simulink model "AircraftSimulation_RealTime1a"  (R2017a)
settings: Solver=ode45  StartTime=0.0  StopTime=inf  RelTol=1e-3  EnableMultiTasking=on
model workspace (MAT data in the model file):
  MCOS : class17 (value not decoded)
values from neighbouring files (symbols this model uses):
  AR = 9.8    [ControlTuning.m]
  b = 12.8016    [ControlTuning.m]
  c = 1.3533    [ControlTuning.m]
  D = d    [rscale.m]
  m = 2521    [ControlTuning.m]
  N = inv([A,B;C,D])*Z'    [rscale.m]
  rho = 0.66    [ControlTuning.m]
  S = 16.72254    [ControlTuning.m]
  s = tf('s')    [ControlTuning.m]    (also in rscale.m = size(A,1))
  W = m*g    (= 24731.01)    [ControlTuning.m]
  Z = [zeros([1,s]) 1]    [rscale.m]
  zeta = Ix*Iz - Ixz^2    (= 5250689.81)    [ControlTuning.m]
undefined symbols (not defined in the file or in its folder): cdo, CLa, ClB, Clda, CLde, Cldr, CLmax, CLo, Clp, CLq, Clr, Cma, Cmde, Cmo, Cmq, CnB, Cnda, Cndr, Cnp, Cnr, CYB, CYda, CYdr, CYp, CYr, da, de, dr, dT, dV_x, dV_y, dV_z, elevation, h, I, Isp, L, mo, mu_e, springK, StallAngle, T, tblackstrip, tControl, tWind, X, xground, xland, Y, yground, yland, ZeroTolerance
libraries: sm_lib x51, nesl_utility x18, simulink x10, realtime_pacer_lib x1
(part 2 of 2)

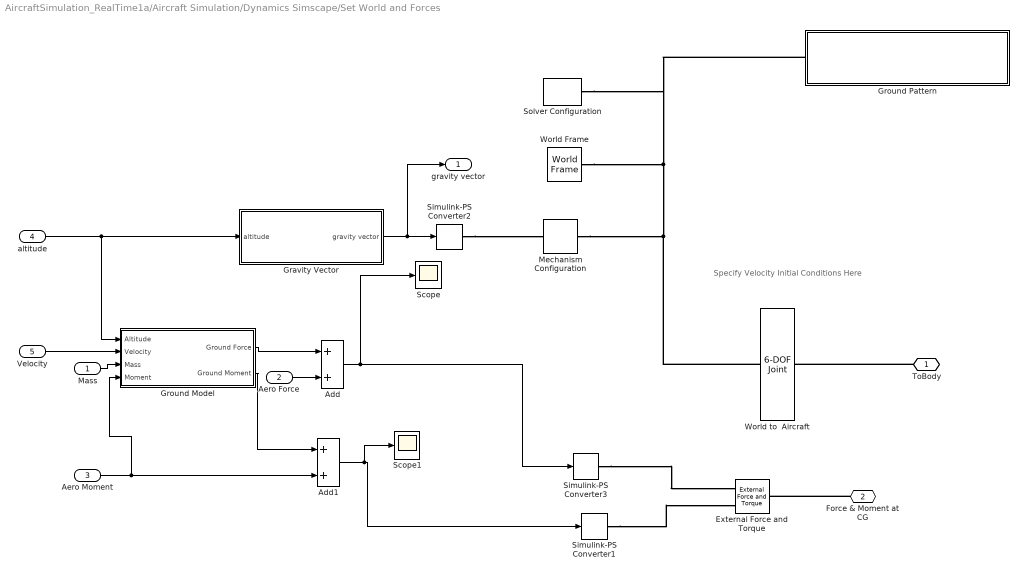
== system AircraftSimulation_RealTime1a/Aircraft Simulation/Dynamics Simscape/Set World and Forces ==
  note: Specify Velocity Initial Conditions Here
  Mass : Inport
  Aero Force : Inport  Port=2
  Aero Moment : Inport  Port=3
  altitude : Inport  Port=4
  Velocity : Inport  Port=5
  Add : Sum
  Add1 : Sum
  External Force and Torque : sm_lib/Forces and Torques/External Force and Torque  ForceResolutionFrame=AttachedFrame  EnableForceX=off  EnableForceY=off  EnableForceZ=off  EnableForce=on  TorqueResolutionFrame=AttachedFrame  EnableTorqueX=off  EnableTorqueY=off  EnableTorqueZ=off  EnableTorque=on
  Gravity Vector : Subsystem
  Ground Model : Subsystem
  Ground Pattern : Subsystem
  Mechanism Configuration : sm_lib/Utilities/Mechanism Configuration  UniformGravity=TimeVarying  GravityVector=[0 0 -9.80665]  GravityUnits=m/s^2  LinearizationDelta=0.001
  Scope : Scope
  Scope1 : Scope
  Simulink-PS Converter1 : nesl_utility/Simulink-PS Converter  PhysicalDomain=network_engine_domain  SubClassName=ps_input  LeftPortType=input  RightPortType=output  PseudoPeriodic=off  Frequencies=[]  NoiseDistribution=none  NoiseParameters=[]  Unit=1  AffineConversion=off  FilteringAndDerivatives=provide  SimscapeFilterOrder=1  InputFilterTimeConstant=0.001  UdotUserProvided=0
  Simulink-PS Converter2 : nesl_utility/Simulink-PS Converter  PhysicalDomain=network_engine_domain  SubClassName=ps_input  LeftPortType=input  RightPortType=output  PseudoPeriodic=off  Frequencies=[]  NoiseDistribution=none  NoiseParameters=[]  Unit=1  AffineConversion=off  FilteringAndDerivatives=provide  SimscapeFilterOrder=1  InputFilterTimeConstant=0.001  UdotUserProvided=0
  Simulink-PS Converter3 : nesl_utility/Simulink-PS Converter  PhysicalDomain=network_engine_domain  SubClassName=ps_input  LeftPortType=input  RightPortType=output  PseudoPeriodic=off  Frequencies=[]  NoiseDistribution=none  NoiseParameters=[]  Unit=1  AffineConversion=off  FilteringAndDerivatives=provide  SimscapeFilterOrder=1  InputFilterTimeConstant=0.001  UdotUserProvided=0
  Solver Configuration : nesl_utility/Solver Configuration  PhysicalDomain=network_engine_domain  SubClassName=solver  LeftPortType=input  RightPortType=generic  Accelerate=off  Tones=[]  Harmonics=[]  SimulateNoise=off  Profile=off  UseLocalSampling=off  EnableSwitchedLinearOptims=on  FrequencyDomain=off  UseCCode=off  RelTol=0.001  AbsTol=1e-06  MinStep=1e-09  ToWorkspace=off  RevertToSquareIcSolve=off  NumHomotopyIterations=100  PhasorMode=off  PhasorModeNumHarmonics=1  OverrideAbsTol=off  DoDC=off  ResidualTolerance=1e-09  UseLocalSolver=off  LocalSolverChoice=NE_BACKWARD_EULER_ADVANCER  LocalSolverSampleTime=0.001  DoFixedCost=off  MaxNonlinIter=3  MaxModeIter=2  LinearAlgebra=Sparse  DelaysMemoryBudget=1024  AutomaticFiltering=on  FilteringTimeConstant=0.001
  World Frame : sm_lib/Frames and Transforms/World Frame
  World to  Aircraft : sm_lib/Joints/6-DOF Joint  SenseConstraintForce=off  SenseConstraintForceX=off  SenseConstraintForceY=off  SenseConstraintForceZ=off  SenseConstraintTorque=off  SenseConstraintTorqueX=off  SenseConstraintTorqueY=off  SenseConstraintTorqueZ=off  SenseTotalForce=off  SenseTotalForceX=off  SenseTotalForceY=off  SenseTotalForceZ=off  SenseTotalTorque=off  SenseTotalTorqueX=off  SenseTotalTorqueY=off  SenseTotalTorqueZ=off  CompositeWrenchDir=BaseOnFollower  CompositeWrenchFrame=BaseFrame  PxEquilibriumPosition=0  PxEquilibriumPositionUnits=m  PxSpringStiffness=0  PxSpringStiffnessUnits=N/m  PxDampingCoefficient=0  PxDampingCoefficientUnits=N/(m/s)  PxTorqueActuationMode=NoTorque  PxMotionActuationMode=ComputedMotion  PxSensePosition=off  PxSenseVelocity=off  PxSenseAcceleration=off  PxSenseTorqueForce=off  PxPositionTargetSpecify=on  PxPositionTargetPriority=High  PxPositionTargetValue=x_initial  PxPositionTargetValueUnits=m  PxVelocityTargetSpecify=on  PxVelocityTargetPriority=High  PxVelocityTargetValue=u_inertial  PxVelocityTargetValueUnits=m/s  PyEquilibriumPosition=0  PyEquilibriumPositionUnits=m  PySpringStiffness=0  PySpringStiffnessUnits=N/m  PyDampingCoefficient=0  PyDampingCoefficientUnits=N/(m/s)  PyTorqueActuationMode=NoTorque  PyMotionActuationMode=ComputedMotion  PySensePosition=off  PySenseVelocity=off  PySenseAcceleration=off  PySenseTorqueForce=off  PyPositionTargetSpecify=on  PyPositionTargetPriority=High  PyPositionTargetValue=y_initial  PyPositionTargetValueUnits=m  PyVelocityTargetSpecify=on  PyVelocityTargetPriority=High  PyVelocityTargetValue=v_inertial  PyVelocityTargetValueUnits=m/s  PzEquilibriumPosition=0  PzEquilibriumPositionUnits=m  PzSpringStiffness=0  PzSpringStiffnessUnits=N/m  PzDampingCoefficient=0  PzDampingCoefficientUnits=N/(m/s)  PzTorqueActuationMode=NoTorque  PzMotionActuationMode=ComputedMotion  PzSensePosition=off  PzSenseVelocity=off  PzSenseAcceleration=off  PzSenseTorqueForce=off  PzPositionTargetSpecify=on  PzPositionTargetPriority=High  PzPositionTargetValue=alt  PzPositionTargetValueUnits=m  PzVelocityTargetSpecify=on  PzVelocityTargetPriority=High  PzVelocityTargetValue=w_inertial  PzVelocityTargetValueUnits=m/s  SphDefPosRotationMethod=None  SphDefPosRotationAngleUnits=deg  SphDefPosRotationStandardAxis=+Z  SphDefPosRotationAngle=0.0  SphDefPosRotationArbitraryAxis=[0 0 1]  SphDefPosFollAlignAxisA=+X  SphDefPosBaseAlignAxisA=+Y  SphDefPosFollAlignAxisB=+Y  SphDefPosBaseAlignAxisB=+Z  SphDefPosRotationSequenceAxes=FollowerAxes  SphDefPosRotationSequence=XYX  SphDefPosRotationSequenceAngles=[0 0 0]  SphDefPosRotationSequenceAnglesUnits=deg  SphDefPosRotationMatrix=[1 0 0; 0 1 0; 0 0 1]  SphEqPosRotationMethod=None  SphEqPosRotationAngleUnits=deg  SphEqPosRotationStandardAxis=+Z  SphEqPosRotationAngle=0.0  SphEqPosRotationArbitraryAxis=[0 0 1]  SphEqPosFollAlignAxisA=+X  SphEqPosBaseAlignAxisA=+Y  SphEqPosFollAlignAxisB=+Y  SphEqPosBaseAlignAxisB=+Z  SphEqPosRotationSequenceAxes=FollowerAxes  SphEqPosRotationSequence=XYX  SphEqPosRotationSequenceAngles=[0 0 0]  SphEqPosRotationSequenceAnglesUnits=deg  SphEqPosRotationMatrix=[1 0 0; 0 1 0; 0 0 1]  SphSpringStiffness=0  SphSpringStiffnessUnits=N*m/deg  SphDampingCoefficient=0  SphDampingCoefficientUnits=N*m/(deg/s)  SphActuateTorqueX=off  SphActuateTorqueY=off  SphActuateTorqueZ=off  SphActuateTorque=on  SphTorqueActuationMode=NoTorque  SphMotionActuationMode=ComputedMotion  SphActuationFrame=BaseFrame  SphSensePosition=off  SphSenseVelocityX=off  SphSenseVelocityY=off  SphSenseVelocityZ=off  SphSenseVelocity=off  SphSenseAccelerationX=off  SphSenseAccelerationY=off  SphSenseAccelerationZ=off  SphSenseAcceleration=off  SphSenseTorqueX=off  SphSenseTorqueY=off  SphSenseTorqueZ=off  SphSenseTorqueForce=off  SphSensingFrame=BaseFrame  SphPositionTargetRotationMethod=StandardAxis  SphPositionTargetRotationAngleUnits=deg  SphPositionTargetRotationStandardAxis=+Y  SphPositionTargetRotationAngle=pitch_initial  SphPositionTargetRotationArbitraryAxis=[0 0 1]  SphPositionTargetFollAlignAxisA=+X  SphPositionTargetBaseAlignAxisA=+Y  SphPositionTargetFollAlignAxisB=+Y  SphPositionTargetBaseAlignAxisB=+Z  SphPositionTargetRotationSequenceAxes=FollowerAxes  SphPositionTargetRotationSequence=XYX  SphPositionTargetRotationSequenceAngles=[0 0 0]  SphPositionTargetRotationSequenceAnglesUnits=deg  SphPositionTargetRotationMatrix=[1 0 0; 0 1 0; 0 0 1]  SphPositionTargetSpecify=on  SphPositionTargetPriority=High  SphVelocityTargetValue=[0 0 0]  SphVelocityTargetValueUnits=deg/s  SphVelocityTargetSpecify=off  SphVelocityTargetPriority=High  SphVelocityTargetInFollowerFrame=on
  ToBody : PMIOPort  Port=1  Side=Right
  Force & Moment at CG : PMIOPort  Port=2  Side=Right
  gravity vector : Outport
  wires:
  Gravity Vector/1(gravity vector) -> gravity vector/1, Simulink-PS Converter2/1
  altitude/1 -> Ground Model/1(Altitude), Gravity Vector/1(altitude)
  Velocity/1 -> Ground Model/2(Velocity)
  Mass/1 -> Ground Model/3(Mass)
  Ground Model/1(Ground Force) -> Add/1
  Aero Force/1 -> Add/2
  Add/1 -> Scope/1, Simulink-PS Converter3/1
  Aero Moment/1 -> Ground Model/4(Moment), Add1/2
  Add1/1 -> Scope1/1, Simulink-PS Converter1/1
  Ground Model/2(Ground Moment) -> Add1/1
  connections:
  Simulink-PS Converter2/RConn1 -- Mechanism Configuration/LConn1
  Ground Pattern/LConn1 -- Solver Configuration/RConn1 -- World to  Aircraft/LConn1 -- Mechanism Configuration/RConn1 -- World Frame/RConn1
  ToBody/RConn1 -- World to  Aircraft/RConn1
  Simulink-PS Converter3/RConn1 -- External Force and Torque/LConn1
  Simulink-PS Converter1/RConn1 -- External Force and Torque/LConn2
  Force & Moment at CG/RConn1 -- External Force and Torque/RConn1

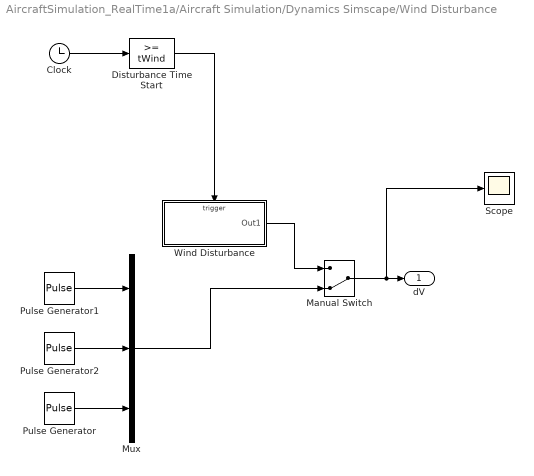
== system AircraftSimulation_RealTime1a/Aircraft Simulation/Dynamics Simscape/Wind Disturbance ==
  Clock : Clock
  Disturbance Time Start : simulink/Logic and Bit Operations/Compare To Constant  relop=>=  const=tWind  OutDataTypeStr=boolean
  Manual Switch : ManualSwitch  CurrentSetting=0
  Mux : Mux  Inputs=3
  Pulse Generator : DiscretePulseGenerator  PulseType=Time based  Amplitude=dV_z  Period=250  PulseWidth=.5  PhaseDelay=5
  Pulse Generator1 : DiscretePulseGenerator  PulseType=Time based  Amplitude=dV_x  Period=250  PulseWidth=.5  PhaseDelay=5
  Pulse Generator2 : DiscretePulseGenerator  PulseType=Time based  Amplitude=dV_y  Period=250  PulseWidth=.5  PhaseDelay=5
  Scope : Scope
  "Wind Disturbance " : Subsystem  TreatAsAtomicUnit=on
  dV : Outport
  wires:
  Clock/1 -> Disturbance Time Start/1
  Disturbance Time Start/1 -> "Wind Disturbance "/Trigger
  Manual Switch/1 -> Scope/1, dV/1
  "Wind Disturbance "/1(Out1) -> Manual Switch/1
  Pulse Generator/1 -> Mux/3
  Mux/1 -> Manual Switch/2
  Pulse Generator2/1 -> Mux/2
  Pulse Generator1/1 -> Mux/1

== system AircraftSimulation_RealTime1a/Aircraft Simulation/Flight Command/Command disturbance ==
  Clock : Clock
  "Cmd Disturbance " : Subsystem  TreatAsAtomicUnit=on
  Disturbance Time Start : simulink/Logic and Bit Operations/Compare To Constant  relop=>=  const=tControl  OutDataTypeStr=boolean
  dCmd : Outport
  wires:
  Clock/1 -> Disturbance Time Start/1
  Disturbance Time Start/1 -> "Cmd Disturbance "/Trigger
  "Cmd Disturbance "/1(Out1) -> dCmd/1

== system AircraftSimulation_RealTime1a/Aircraft Simulation/Aerodynamics Simscape/Forces and Moments/Small Number = Zero6 ==
  In1 : Inport
  Abs : Abs
  Compare To Constant : simulink/Logic and Bit Operations/Compare To Constant  relop=>=  const=ZeroTolerance  OutDataTypeStr=boolean
  Product1 : Product  Inputs=3
  Sign : Signum
  Out1 : Outport
  wires:
  Sign/1 -> Product1/3
  Abs/1 -> Compare To Constant/1, Product1/1
  Product1/1 -> Out1/1
  Compare To Constant/1 -> Product1/2
  In1/1 -> Abs/1, Sign/1

== system AircraftSimulation_RealTime1a/Aircraft Simulation/Aerodynamics Simscape/Forces and Moments/Stall ==
  In1 : Inport
  Abs : Abs
  Compare To Constant : simulink/Logic and Bit Operations/Compare To Constant  relop=>  const=StallAngle  OutDataTypeStr=boolean
  Demux : Demux
  Terminator : Terminator
  Terminator1 : Terminator
  Terminator2 : Terminator
  Stall : Outport
  wires:
  Demux/3 -> Terminator1/1
  Demux/4 -> Terminator2/1
  Demux/2 -> Abs/1
  Demux/1 -> Terminator/1
  Compare To Constant/1 -> Stall/1
  In1/1 -> Demux/1
  Abs/1 -> Compare To Constant/1

== system AircraftSimulation_RealTime1a/Aircraft Simulation/Aerodynamics Simscape/Forces and Moments/stall effect ==
  lift : Inport
  stall : Inport  Port=2
  Compare To Constant : simulink/Logic and Bit Operations/Compare To Constant  relop=<=  const=1  OutDataTypeStr=boolean
  Product1 : Product
  Lift : Outport
  wires:
  lift/1 -> Product1/1
  Compare To Constant/1 -> Product1/2
  stall/1 -> Compare To Constant/1
  Product1/1 -> Lift/1

== system AircraftSimulation_RealTime1a/Aircraft Simulation/Aerodynamics Simscape/Forces and Moments/stall effect1 ==
  moment : Inport
  stall : Inport  Port=2
  Compare To Constant : simulink/Logic and Bit Operations/Compare To Constant  relop=<=  const=1  OutDataTypeStr=boolean
  Product1 : Product
  Moment : Outport
  wires:
  Product1/1 -> Moment/1
  stall/1 -> Compare To Constant/1
  Compare To Constant/1 -> Product1/2
  moment/1 -> Product1/1

== system AircraftSimulation_RealTime1a/Aircraft Simulation/Dynamics Simscape/Derived States/Cannot Divide By Zero ==
  Denominator In : Inport
  Else Action Subsystem : Subsystem  TreatAsAtomicUnit=on
  If : If  IfExpression=u1 == 0
  "If Action Subsystem " : Subsystem  TreatAsAtomicUnit=on
  Merge : Merge
  Denominator Out : Outport
  wires:
  Denominator In/1 -> Else Action Subsystem/1(In1), If/1
  "If Action Subsystem "/1(Out1) -> Merge/1
  If/1 -> "If Action Subsystem "/Action
  If/2 -> Else Action Subsystem/Action
  Else Action Subsystem/1(Out1) -> Merge/2
  Merge/1 -> Denominator Out/1

== system AircraftSimulation_RealTime1a/Aircraft Simulation/Dynamics Simscape/Derived States/Cannot Divide By Zero1 ==
  Denominator In : Inport
  Else Action Subsystem : Subsystem  TreatAsAtomicUnit=on
  If : If  IfExpression=u1 == 0
  "If Action Subsystem " : Subsystem  TreatAsAtomicUnit=on
  Merge : Merge
  Denominator Out : Outport
  wires:
  Merge/1 -> Denominator Out/1
  Else Action Subsystem/1(Out1) -> Merge/2
  If/2 -> Else Action Subsystem/Action
  If/1 -> "If Action Subsystem "/Action
  "If Action Subsystem "/1(Out1) -> Merge/1
  Denominator In/1 -> If/1, Else Action Subsystem/1(In1)

== system AircraftSimulation_RealTime1a/Aircraft Simulation/Dynamics Simscape/Derived States/Magnitude ==
  Vector : Inport
  Demux : Demux  Outputs=3
  Product1 : Product
  Product2 : Product
  Product3 : Product
  Sqrt : Sqrt  SaturateOnIntegerOverflow=on
  Sum : Sum  Inputs=+++
  Magnitude : Outport
  wires:
  Demux/1 -> Product1/1, Product1/2
  Demux/3 -> Product3/1, Product3/2
  Product2/1 -> Sum/2
  Product1/1 -> Sum/1
  Sum/1 -> Sqrt/1
  Demux/2 -> Product2/1, Product2/2
  Product3/1 -> Sum/3
  Vector/1 -> Demux/1
  Sqrt/1 -> Magnitude/1

== system AircraftSimulation_RealTime1a/Aircraft Simulation/Dynamics Simscape/Derived States/Small Number = Zero1 ==
  In1 : Inport
  Abs : Abs
  Compare To Constant : simulink/Logic and Bit Operations/Compare To Constant  relop=>=  const=ZeroTolerance  OutDataTypeStr=boolean
  Product1 : Product  Inputs=3
  Sign : Signum
  Out1 : Outport
  wires:
  In1/1 -> Sign/1, Abs/1
  Compare To Constant/1 -> Product1/2
  Product1/1 -> Out1/1
  Abs/1 -> Product1/1, Compare To Constant/1
  Sign/1 -> Product1/3

== system AircraftSimulation_RealTime1a/Aircraft Simulation/Dynamics Simscape/Derived States/Small Number = Zero2 ==
  In1 : Inport
  Abs : Abs
  Compare To Constant : simulink/Logic and Bit Operations/Compare To Constant  relop=>=  const=ZeroTolerance  OutDataTypeStr=boolean
  Product1 : Product  Inputs=3
  Sign : Signum
  Out1 : Outport
  wires:
  In1/1 -> Sign/1, Abs/1
  Compare To Constant/1 -> Product1/2
  Product1/1 -> Out1/1
  Abs/1 -> Product1/1, Compare To Constant/1
  Sign/1 -> Product1/3

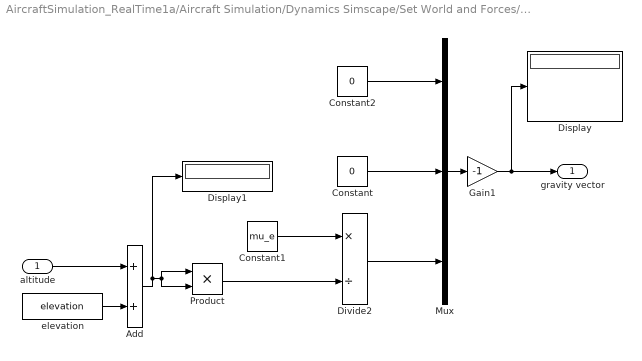
== system AircraftSimulation_RealTime1a/Aircraft Simulation/Dynamics Simscape/Set World and Forces/Gravity Vector ==
  altitude : Inport
  Add : Sum
  Constant : Constant  Value=0
  Constant1 : Constant  Value=mu_e
  Constant2 : Constant  Value=0
  Display : Display
  Display1 : Display
  Divide2 : Product  Inputs=*/
  Gain1 : Gain  Gain=-1
  Mux : Mux  Inputs=3
  Product : Product
  elevation : Constant  Value=elevation
  gravity vector : Outport
  wires:
  Constant1/1 -> Divide2/1
  Constant/1 -> Mux/2
  Product/1 -> Divide2/2
  Add/1 -> Display1/1, Product/1, Product/2
  elevation/1 -> Add/2
  Constant2/1 -> Mux/1
  Mux/1 -> Gain1/1
  Divide2/1 -> Mux/3
  altitude/1 -> Add/1
  Gain1/1 -> Display/1, gravity vector/1

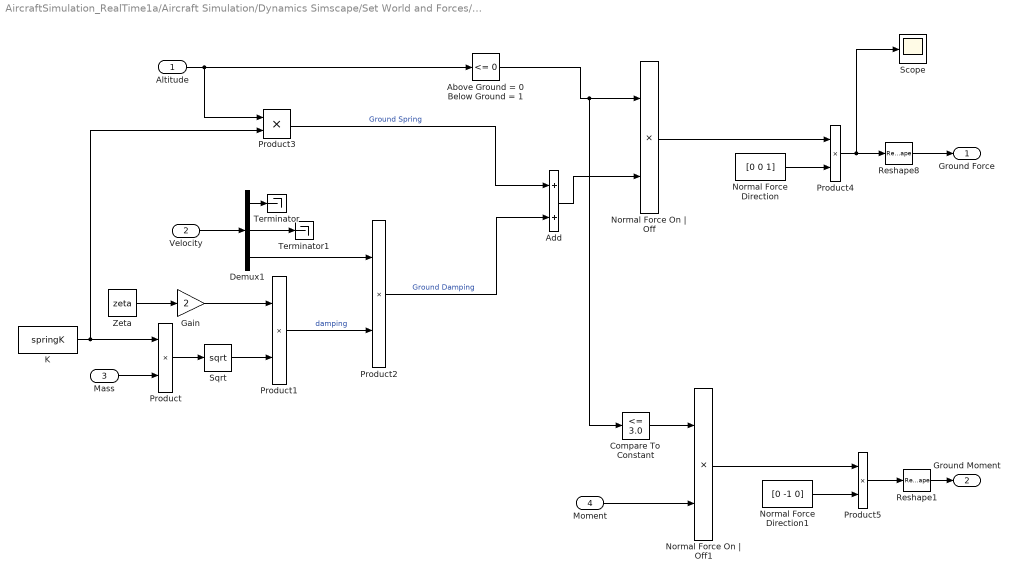
== system AircraftSimulation_RealTime1a/Aircraft Simulation/Dynamics Simscape/Set World and Forces/Ground Model ==
  Altitude : Inport
  Velocity : Inport  Port=2
  Mass : Inport  Port=3
  Moment : Inport  Port=4
  Above Ground = 0 Below Ground = 1 : simulink/Logic and Bit Operations/Compare To Zero  relop=<=  OutDataTypeStr=boolean
  Add : Sum
  Compare To Constant : simulink/Logic and Bit Operations/Compare To Constant  relop=<=  const=3.0  OutDataTypeStr=boolean
  Demux1 : Demux  Outputs=3
  Gain : Gain  Gain=2
  K : Constant  Value=springK
  Normal Force Direction : Constant  Value=[0 0 1]
  Normal Force Direction1 : Constant  Value=[0 -1 0]
  Normal Force On | Off : Product
  Normal Force On | Off1 : Product
  Product{,1..5} (6 alike) : Product
  Reshape1 : Reshape  OutputDimensionality=Column vector (2-D)
  Reshape8 : Reshape  OutputDimensionality=Column vector (2-D)
  Scope : Scope
  Sqrt : Sqrt  SaturateOnIntegerOverflow=on
  Terminator : Terminator
  Terminator1 : Terminator
  Zeta : Constant  Value=zeta
  Ground Force : Outport
  Ground Moment : Outport  Port=2
  wires:
  Velocity/1 -> Demux1/1
  Demux1/1 -> Terminator/1
  Altitude/1 -> Product3/1, Above Ground = 0 Below Ground = 1/1
  Demux1/2 -> Terminator1/1
  Above Ground = 0 Below Ground = 1/1 -> Compare To Constant/1, Normal Force On | Off/1
  Zeta/1 -> Gain/1
  Product/1 -> Sqrt/1
  Gain/1 -> Product1/1
  Sqrt/1 -> Product1/2
  Demux1/3 -> Product2/1
  Product1/1 -> Product2/2  "damping"
  K/1 -> Product3/2, Product/1
  Mass/1 -> Product/2
  Add/1 -> Normal Force On | Off/2
  Product3/1 -> Add/1  "Ground Spring"
  Product2/1 -> Add/2  "Ground Damping"
  Reshape8/1 -> Ground Force/1
  Product4/1 -> Scope/1, Reshape8/1
  Normal Force Direction/1 -> Product4/2
  Normal Force On | Off/1 -> Product4/1
  Compare To Constant/1 -> Normal Force On | Off1/1
  Normal Force Direction1/1 -> Product5/2
  Normal Force On | Off1/1 -> Product5/1
  Product5/1 -> Reshape1/1
  Reshape1/1 -> Ground Moment/1
  Moment/1 -> Normal Force On | Off1/2

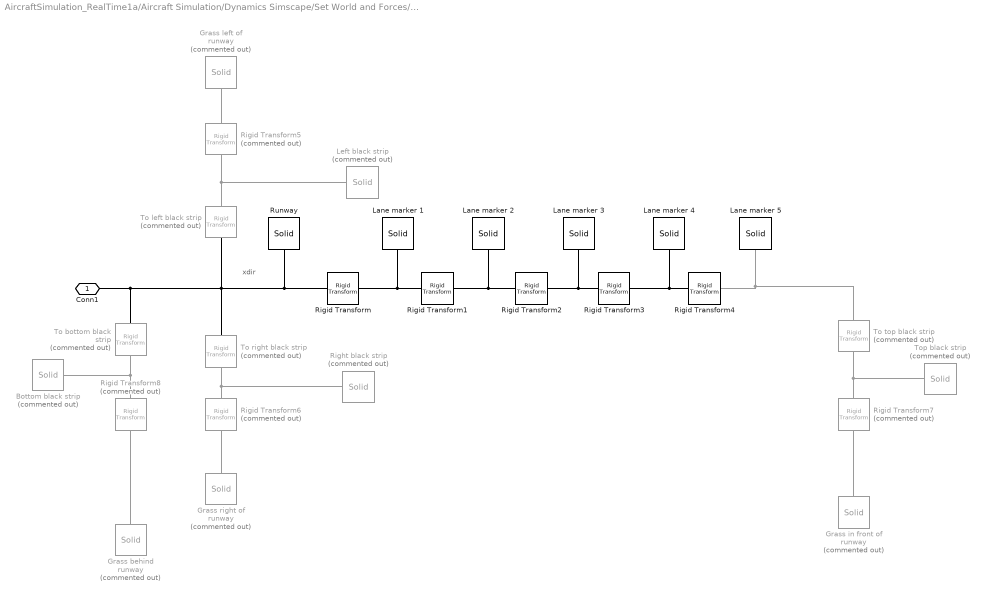
== system AircraftSimulation_RealTime1a/Aircraft Simulation/Dynamics Simscape/Set World and Forces/Ground Pattern ==
  note: xdir
  Bottom black strip : sm_lib/Body Elements/Solid  Commented=on  InertiaType=CalculateFromGeometry  Mass=1  MassUnits=kg  CenterOfMass=[0 0 0]  CenterOfMassUnits=m  MomentsOfInertia=[1 1 1]  MomentsOfInertiaUnits=kg*m^2  ProductsOfInertia=[1 1 1]  ProductsOfInertiaUnits=kg*m^2  DensityBased=on  Density=1000  DensityUnits=kg/m^3  DoExposeReferenceFrame=on  SerializedFrames=<Frames/>  GraphicType=FromGeometry  MarkerShape=Sphere  MarkerSize=10  GraphicVisPropType=SimpleVisualProperties  GraphicDiffuseColor=[0.0 0.0 0.0]  GraphicSpecularColor=[0.5 0.5 0.5 1.0]  GraphicAmbientColor=[0.15 0.15 0.15 1.0]  GraphicEmissiveColor=[0.0 0.0 0.0 1.0]  GraphicShininess=75  GraphicOpacity=1.0  GeometryShape=Brick  RectangleSize=[1 1]  RectangleSizeUnits=m  BrickDimensions=[tblackstrip, yland, 0.1]  BrickDimensionUnits=m  CylinderRadius=1  CylinderRadiusUnits=m  CylinderLength=1  CylinderLengthUnits=m  SphereRadius=1  SphereRadiusUnits=m  EllipsoidRadii=[1 1 1]  EllipsoidRadiiUnits=m  ExtrusionCrossSection=[1 1; -1 1; -1 -1; 1 -1]  ExtrusionCrossSectionUnits=m  ExtrusionLength=1  ExtrusionLengthUnits=m  PolygonNumSides=3  PolygonOuterRadius=1  PolygonOuterRadiusUnits=m  ExtGeomFileType=STEP  ExtGeomFileUnits=m  RevolutionCrossSection=[1 1; 1 -1; 2 -1; 2 1]  RevolutionCrossSectionUnits=m  RevolutionExtent=Full  RevolutionAngle=180  RevolutionAngleUnits=deg
  Grass behind runway : sm_lib/Body Elements/Solid  Commented=on  InertiaType=CalculateFromGeometry  Mass=1  MassUnits=kg  CenterOfMass=[0 0 0]  CenterOfMassUnits=m  MomentsOfInertia=[1 1 1]  MomentsOfInertiaUnits=kg*m^2  ProductsOfInertia=[1 1 1]  ProductsOfInertiaUnits=kg*m^2  DensityBased=on  Density=1000  DensityUnits=kg/m^3  DoExposeReferenceFrame=on  SerializedFrames=<Frames/>  GraphicType=FromGeometry  MarkerShape=Sphere  MarkerSize=10  GraphicVisPropType=SimpleVisualProperties  GraphicDiffuseColor=[0.0 1.0 0.0]  GraphicSpecularColor=[0.5 0.5 0.5 1.0]  GraphicAmbientColor=[0.15 0.15 0.15 1.0]  GraphicEmissiveColor=[0.0 0.0 0.0 1.0]  GraphicShininess=75  GraphicOpacity=1.0  GeometryShape=Brick  RectangleSize=[1 1]  RectangleSizeUnits=m  BrickDimensions=[2*xground, 2*yground+yland, 0.1]  BrickDimensionUnits=m  CylinderRadius=1  CylinderRadiusUnits=m  CylinderLength=1  CylinderLengthUnits=m  SphereRadius=1  SphereRadiusUnits=m  EllipsoidRadii=[1 1 1]  EllipsoidRadiiUnits=m  ExtrusionCrossSection=[1 1; -1 1; -1 -1; 1 -1]  ExtrusionCrossSectionUnits=m  ExtrusionLength=1  ExtrusionLengthUnits=m  PolygonNumSides=3  PolygonOuterRadius=1  PolygonOuterRadiusUnits=m  ExtGeomFileType=STEP  ExtGeomFileUnits=m  RevolutionCrossSection=[1 1; 1 -1; 2 -1; 2 1]  RevolutionCrossSectionUnits=m  RevolutionExtent=Full  RevolutionAngle=180  RevolutionAngleUnits=deg
  Grass in front of runway : sm_lib/Body Elements/Solid  Commented=on  InertiaType=CalculateFromGeometry  Mass=1  MassUnits=kg  CenterOfMass=[0 0 0]  CenterOfMassUnits=m  MomentsOfInertia=[1 1 1]  MomentsOfInertiaUnits=kg*m^2  ProductsOfInertia=[1 1 1]  ProductsOfInertiaUnits=kg*m^2  DensityBased=on  Density=1000  DensityUnits=kg/m^3  DoExposeReferenceFrame=on  SerializedFrames=<Frames/>  GraphicType=FromGeometry  MarkerShape=Sphere  MarkerSize=10  GraphicVisPropType=SimpleVisualProperties  GraphicDiffuseColor=[0.0 1.0 0.0]  GraphicSpecularColor=[0.5 0.5 0.5 1.0]  GraphicAmbientColor=[0.15 0.15 0.15 1.0]  GraphicEmissiveColor=[0.0 0.0 0.0 1.0]  GraphicShininess=75  GraphicOpacity=1.0  GeometryShape=Brick  RectangleSize=[1 1]  RectangleSizeUnits=m  BrickDimensions=[2*xground, 2*yground+yland, 0.1]  BrickDimensionUnits=m  CylinderRadius=1  CylinderRadiusUnits=m  CylinderLength=1  CylinderLengthUnits=m  SphereRadius=1  SphereRadiusUnits=m  EllipsoidRadii=[1 1 1]  EllipsoidRadiiUnits=m  ExtrusionCrossSection=[1 1; -1 1; -1 -1; 1 -1]  ExtrusionCrossSectionUnits=m  ExtrusionLength=1  ExtrusionLengthUnits=m  PolygonNumSides=3  PolygonOuterRadius=1  PolygonOuterRadiusUnits=m  ExtGeomFileType=STEP  ExtGeomFileUnits=m  RevolutionCrossSection=[1 1; 1 -1; 2 -1; 2 1]  RevolutionCrossSectionUnits=m  RevolutionExtent=Full  RevolutionAngle=180  RevolutionAngleUnits=deg
  Grass left of runway : sm_lib/Body Elements/Solid  Commented=on  InertiaType=CalculateFromGeometry  Mass=1  MassUnits=kg  CenterOfMass=[0 0 0]  CenterOfMassUnits=m  MomentsOfInertia=[1 1 1]  MomentsOfInertiaUnits=kg*m^2  ProductsOfInertia=[1 1 1]  ProductsOfInertiaUnits=kg*m^2  DensityBased=on  Density=1000  DensityUnits=kg/m^3  DoExposeReferenceFrame=on  SerializedFrames=<Frames/>  GraphicType=FromGeometry  MarkerShape=Sphere  MarkerSize=10  GraphicVisPropType=SimpleVisualProperties  GraphicDiffuseColor=[0.0 1.0 0.0]  GraphicSpecularColor=[0.5 0.5 0.5 1.0]  GraphicAmbientColor=[0.15 0.15 0.15 1.0]  GraphicEmissiveColor=[0.0 0.0 0.0 1.0]  GraphicShininess=75  GraphicOpacity=1.0  GeometryShape=Brick  RectangleSize=[1 1]  RectangleSizeUnits=m  BrickDimensions=[xland yground 0.1]  BrickDimensionUnits=m  CylinderRadius=1  CylinderRadiusUnits=m  CylinderLength=1  CylinderLengthUnits=m  SphereRadius=1  SphereRadiusUnits=m  EllipsoidRadii=[1 1 1]  EllipsoidRadiiUnits=m  ExtrusionCrossSection=[1 1; -1 1; -1 -1; 1 -1]  ExtrusionCrossSectionUnits=m  ExtrusionLength=1  ExtrusionLengthUnits=m  PolygonNumSides=3  PolygonOuterRadius=1  PolygonOuterRadiusUnits=m  ExtGeomFileType=STEP  ExtGeomFileUnits=m  RevolutionCrossSection=[1 1; 1 -1; 2 -1; 2 1]  RevolutionCrossSectionUnits=m  RevolutionExtent=Full  RevolutionAngle=180  RevolutionAngleUnits=deg
  Grass right of runway : sm_lib/Body Elements/Solid  Commented=on  InertiaType=CalculateFromGeometry  Mass=1  MassUnits=kg  CenterOfMass=[0 0 0]  CenterOfMassUnits=m  MomentsOfInertia=[1 1 1]  MomentsOfInertiaUnits=kg*m^2  ProductsOfInertia=[1 1 1]  ProductsOfInertiaUnits=kg*m^2  DensityBased=on  Density=1000  DensityUnits=kg/m^3  DoExposeReferenceFrame=on  SerializedFrames=<Frames/>  GraphicType=FromGeometry  MarkerShape=Sphere  MarkerSize=10  GraphicVisPropType=SimpleVisualProperties  GraphicDiffuseColor=[0.0 1.0 0.0]  GraphicSpecularColor=[0.5 0.5 0.5 1.0]  GraphicAmbientColor=[0.15 0.15 0.15 1.0]  GraphicEmissiveColor=[0.0 0.0 0.0 1.0]  GraphicShininess=75  GraphicOpacity=1.0  GeometryShape=Brick  RectangleSize=[1 1]  RectangleSizeUnits=m  BrickDimensions=[xland yground 0.1]  BrickDimensionUnits=m  CylinderRadius=1  CylinderRadiusUnits=m  CylinderLength=1  CylinderLengthUnits=m  SphereRadius=1  SphereRadiusUnits=m  EllipsoidRadii=[1 1 1]  EllipsoidRadiiUnits=m  ExtrusionCrossSection=[1 1; -1 1; -1 -1; 1 -1]  ExtrusionCrossSectionUnits=m  ExtrusionLength=1  ExtrusionLengthUnits=m  PolygonNumSides=3  PolygonOuterRadius=1  PolygonOuterRadiusUnits=m  ExtGeomFileType=STEP  ExtGeomFileUnits=m  RevolutionCrossSection=[1 1; 1 -1; 2 -1; 2 1]  RevolutionCrossSectionUnits=m  RevolutionExtent=Full  RevolutionAngle=180  RevolutionAngleUnits=deg
  Lane marker {1..5} (5 alike) : sm_lib/Body Elements/Solid  InertiaType=CalculateFromGeometry  Mass=1  MassUnits=kg  CenterOfMass=[0 0 0]  CenterOfMassUnits=m  MomentsOfInertia=[1 1 1]  MomentsOfInertiaUnits=kg*m^2  ProductsOfInertia=[1 1 1]  ProductsOfInertiaUnits=kg*m^2  DensityBased=on  Density=1000  DensityUnits=kg/m^3  DoExposeReferenceFrame=on  SerializedFrames=<Frames/>  GraphicType=FromGeometry  MarkerShape=Sphere  MarkerSize=10  GraphicVisPropType=SimpleVisualProperties  GraphicDiffuseColor=[1.0 1.0 1.0]  GraphicSpecularColor=[0.5 0.5 0.5 1.0]  GraphicAmbientColor=[0.15 0.15 0.15 1.0]  GraphicEmissiveColor=[0.0 0.0 0.0 1.0]  GraphicShininess=75  GraphicOpacity=1.0  GeometryShape=Brick  RectangleSize=[1 1]  RectangleSizeUnits=m  BrickDimensions=[xland/10 yland/10 0.1]  BrickDimensionUnits=m  CylinderRadius=1  CylinderRadiusUnits=m  CylinderLength=1  CylinderLengthUnits=m  SphereRadius=1  SphereRadiusUnits=m  EllipsoidRadii=[1 1 1]  EllipsoidRadiiUnits=m  ExtrusionCrossSection=[1 1; -1 1; -1 -1; 1 -1]  ExtrusionCrossSectionUnits=m  ExtrusionLength=1  ExtrusionLengthUnits=m  PolygonNumSides=3  PolygonOuterRadius=1  PolygonOuterRadiusUnits=m  ExtGeomFileType=STEP  ExtGeomFileUnits=m  RevolutionCrossSection=[1 1; 1 -1; 2 -1; 2 1]  RevolutionCrossSectionUnits=m  RevolutionExtent=Full  RevolutionAngle=180  RevolutionAngleUnits=deg
  Left black strip : sm_lib/Body Elements/Solid  Commented=on  InertiaType=CalculateFromGeometry  Mass=1  MassUnits=kg  CenterOfMass=[0 0 0]  CenterOfMassUnits=m  MomentsOfInertia=[1 1 1]  MomentsOfInertiaUnits=kg*m^2  ProductsOfInertia=[1 1 1]  ProductsOfInertiaUnits=kg*m^2  DensityBased=on  Density=1000  DensityUnits=kg/m^3  DoExposeReferenceFrame=on  SerializedFrames=<Frames/>  GraphicType=FromGeometry  MarkerShape=Sphere  MarkerSize=10  GraphicVisPropType=SimpleVisualProperties  GraphicDiffuseColor=[0.0 0.0 0.0]  GraphicSpecularColor=[0.5 0.5 0.5 1.0]  GraphicAmbientColor=[0.15 0.15 0.15 1.0]  GraphicEmissiveColor=[0.0 0.0 0.0 1.0]  GraphicShininess=75  GraphicOpacity=1.0  GeometryShape=Brick  RectangleSize=[1 1]  RectangleSizeUnits=m  BrickDimensions=[xland, tblackstrip, 0.1]  BrickDimensionUnits=m  CylinderRadius=1  CylinderRadiusUnits=m  CylinderLength=1  CylinderLengthUnits=m  SphereRadius=1  SphereRadiusUnits=m  EllipsoidRadii=[1 1 1]  EllipsoidRadiiUnits=m  ExtrusionCrossSection=[1 1; -1 1; -1 -1; 1 -1]  ExtrusionCrossSectionUnits=m  ExtrusionLength=1  ExtrusionLengthUnits=m  PolygonNumSides=3  PolygonOuterRadius=1  PolygonOuterRadiusUnits=m  ExtGeomFileType=STEP  ExtGeomFileUnits=m  RevolutionCrossSection=[1 1; 1 -1; 2 -1; 2 1]  RevolutionCrossSectionUnits=m  RevolutionExtent=Full  RevolutionAngle=180  RevolutionAngleUnits=deg
  Right black strip : sm_lib/Body Elements/Solid  Commented=on  InertiaType=CalculateFromGeometry  Mass=1  MassUnits=kg  CenterOfMass=[0 0 0]  CenterOfMassUnits=m  MomentsOfInertia=[1 1 1]  MomentsOfInertiaUnits=kg*m^2  ProductsOfInertia=[1 1 1]  ProductsOfInertiaUnits=kg*m^2  DensityBased=on  Density=1000  DensityUnits=kg/m^3  DoExposeReferenceFrame=on  SerializedFrames=<Frames/>  GraphicType=FromGeometry  MarkerShape=Sphere  MarkerSize=10  GraphicVisPropType=SimpleVisualProperties  GraphicDiffuseColor=[0.0 0.0 0.0]  GraphicSpecularColor=[0.5 0.5 0.5 1.0]  GraphicAmbientColor=[0.15 0.15 0.15 1.0]  GraphicEmissiveColor=[0.0 0.0 0.0 1.0]  GraphicShininess=75  GraphicOpacity=1.0  GeometryShape=Brick  RectangleSize=[1 1]  RectangleSizeUnits=m  BrickDimensions=[xland, tblackstrip, 0.1]  BrickDimensionUnits=m  CylinderRadius=1  CylinderRadiusUnits=m  CylinderLength=1  CylinderLengthUnits=m  SphereRadius=1  SphereRadiusUnits=m  EllipsoidRadii=[1 1 1]  EllipsoidRadiiUnits=m  ExtrusionCrossSection=[1 1; -1 1; -1 -1; 1 -1]  ExtrusionCrossSectionUnits=m  ExtrusionLength=1  ExtrusionLengthUnits=m  PolygonNumSides=3  PolygonOuterRadius=1  PolygonOuterRadiusUnits=m  ExtGeomFileType=STEP  ExtGeomFileUnits=m  RevolutionCrossSection=[1 1; 1 -1; 2 -1; 2 1]  RevolutionCrossSectionUnits=m  RevolutionExtent=Full  RevolutionAngle=180  RevolutionAngleUnits=deg
  Rigid Transform : sm_lib/Frames and Transforms/Rigid Transform  TranslationMethod=Cartesian  TranslationStandardOffset=0  TranslationLengthUnit=m  TranslationStandardAxis=+Z  TranslationCartesianOffset=[-xland/2 + xland/10 0 0.1]  TranslationROffset=0  TranslationROffsetUnits=m  TranslationZOffset=0  TranslationZOffsetUnits=m  TranslationThetaOffset=0  TranslationThetaOffsetUnits=deg  RotationMethod=None  RotationAngleUnits=deg  RotationStandardAxis=+Z  RotationAngle=0.0  RotationArbitraryAxis=[0 0 1]  FollAlignAxisA=+X  BaseAlignAxisA=+Y  FollAlignAxisB=+Y  BaseAlignAxisB=+Z  RotationSequenceAxes=FollowerAxes  RotationSequence=XYX  RotationSequenceAngles=[0 0 0]  RotationSequenceAnglesUnits=deg  RotationMatrix=[1 0 0; 0 1 0; 0 0 1]
  Rigid Transform{1..4} (4 alike) : sm_lib/Frames and Transforms/Rigid Transform  TranslationMethod=Cartesian  TranslationStandardOffset=0  TranslationLengthUnit=m  TranslationStandardAxis=+Z  TranslationCartesianOffset=[xland/5 0 0]  TranslationROffset=0  TranslationROffsetUnits=m  TranslationZOffset=0  TranslationZOffsetUnits=m  TranslationThetaOffset=0  TranslationThetaOffsetUnits=deg  RotationMethod=None  RotationAngleUnits=deg  RotationStandardAxis=+Z  RotationAngle=0.0  RotationArbitraryAxis=[0 0 1]  FollAlignAxisA=+X  BaseAlignAxisA=+Y  FollAlignAxisB=+Y  BaseAlignAxisB=+Z  RotationSequenceAxes=FollowerAxes  RotationSequence=XYX  RotationSequenceAngles=[0 0 0]  RotationSequenceAnglesUnits=deg  RotationMatrix=[1 0 0; 0 1 0; 0 0 1]
  Rigid Transform5 : sm_lib/Frames and Transforms/Rigid Transform  Commented=on  TranslationMethod=Cartesian  TranslationStandardOffset=0  TranslationLengthUnit=m  TranslationStandardAxis=+Z  TranslationCartesianOffset=[0, yland/2+tblackstrip, 0]  TranslationROffset=0  TranslationROffsetUnits=m  TranslationZOffset=0  TranslationZOffsetUnits=m  TranslationThetaOffset=0  TranslationThetaOffsetUnits=deg  RotationMethod=None  RotationAngleUnits=deg  RotationStandardAxis=+Z  RotationAngle=0.0  RotationArbitraryAxis=[0 0 1]  FollAlignAxisA=+X  BaseAlignAxisA=+Y  FollAlignAxisB=+Y  BaseAlignAxisB=+Z  RotationSequenceAxes=FollowerAxes  RotationSequence=XYX  RotationSequenceAngles=[0 0 0]  RotationSequenceAnglesUnits=deg  RotationMatrix=[1 0 0; 0 1 0; 0 0 1]
  Rigid Transform6 : sm_lib/Frames and Transforms/Rigid Transform  Commented=on  TranslationMethod=Cartesian  TranslationStandardOffset=0  TranslationLengthUnit=m  TranslationStandardAxis=+Z  TranslationCartesianOffset=[0, tblackstrip, 0]  TranslationROffset=0  TranslationROffsetUnits=m  TranslationZOffset=0  TranslationZOffsetUnits=m  TranslationThetaOffset=0  TranslationThetaOffsetUnits=deg  RotationMethod=None  RotationAngleUnits=deg  RotationStandardAxis=+Z  RotationAngle=0.0  RotationArbitraryAxis=[0 0 1]  FollAlignAxisA=+X  BaseAlignAxisA=+Y  FollAlignAxisB=+Y  BaseAlignAxisB=+Z  RotationSequenceAxes=FollowerAxes  RotationSequence=XYX  RotationSequenceAngles=[0 0 0]  RotationSequenceAnglesUnits=deg  RotationMatrix=[1 0 0; 0 1 0; 0 0 1]
  Rigid Transform7 : sm_lib/Frames and Transforms/Rigid Transform  Commented=on  TranslationMethod=Cartesian  TranslationStandardOffset=0  TranslationLengthUnit=m  TranslationStandardAxis=+Z  TranslationCartesianOffset=[tblackstrip, 0, 0]  TranslationROffset=0  TranslationROffsetUnits=m  TranslationZOffset=0  TranslationZOffsetUnits=m  TranslationThetaOffset=0  TranslationThetaOffsetUnits=deg  RotationMethod=None  RotationAngleUnits=deg  RotationStandardAxis=+Z  RotationAngle=0.0  RotationArbitraryAxis=[0 0 1]  FollAlignAxisA=+X  BaseAlignAxisA=+Y  FollAlignAxisB=+Y  BaseAlignAxisB=+Z  RotationSequenceAxes=FollowerAxes  RotationSequence=XYX  RotationSequenceAngles=[0 0 0]  RotationSequenceAnglesUnits=deg  RotationMatrix=[1 0 0; 0 1 0; 0 0 1]
  Rigid Transform8 : sm_lib/Frames and Transforms/Rigid Transform  Commented=on  TranslationMethod=Cartesian  TranslationStandardOffset=0  TranslationLengthUnit=m  TranslationStandardAxis=+Z  TranslationCartesianOffset=[-tblackstrip, 0, 0]  TranslationROffset=0  TranslationROffsetUnits=m  TranslationZOffset=0  TranslationZOffsetUnits=m  TranslationThetaOffset=0  TranslationThetaOffsetUnits=deg  RotationMethod=None  RotationAngleUnits=deg  RotationStandardAxis=+Z  RotationAngle=0.0  RotationArbitraryAxis=[0 0 1]  FollAlignAxisA=+X  BaseAlignAxisA=+Y  FollAlignAxisB=+Y  BaseAlignAxisB=+Z  RotationSequenceAxes=FollowerAxes  RotationSequence=XYX  RotationSequenceAngles=[0 0 0]  RotationSequenceAnglesUnits=deg  RotationMatrix=[1 0 0; 0 1 0; 0 0 1]
  Runway : sm_lib/Body Elements/Solid  InertiaType=CalculateFromGeometry  Mass=1  MassUnits=kg  CenterOfMass=[0 0 0]  CenterOfMassUnits=m  MomentsOfInertia=[1 1 1]  MomentsOfInertiaUnits=kg*m^2  ProductsOfInertia=[1 1 1]  ProductsOfInertiaUnits=kg*m^2  DensityBased=on  Density=1000  DensityUnits=kg/m^3  DoExposeReferenceFrame=on  SerializedFrames=<Frames/>  GraphicType=FromGeometry  MarkerShape=Sphere  MarkerSize=10  GraphicVisPropType=SimpleVisualProperties  GraphicDiffuseColor=[0.8 0.8 0.8]  GraphicSpecularColor=[0.5 0.5 0.5 1.0]  GraphicAmbientColor=[0.15 0.15 0.15 1.0]  GraphicEmissiveColor=[0.0 0.0 0.0 1.0]  GraphicShininess=75  GraphicOpacity=1.0  GeometryShape=Brick  RectangleSize=[1 1]  RectangleSizeUnits=m  BrickDimensions=[xland yland 0.1]  BrickDimensionUnits=m  CylinderRadius=1  CylinderRadiusUnits=m  CylinderLength=1  CylinderLengthUnits=m  SphereRadius=1  SphereRadiusUnits=m  EllipsoidRadii=[1 1 1]  EllipsoidRadiiUnits=m  ExtrusionCrossSection=[1 1; -1 1; -1 -1; 1 -1]  ExtrusionCrossSectionUnits=m  ExtrusionLength=1  ExtrusionLengthUnits=m  PolygonNumSides=3  PolygonOuterRadius=1  PolygonOuterRadiusUnits=m  ExtGeomFileType=STEP  ExtGeomFileUnits=m  RevolutionCrossSection=[1 1; 1 -1; 2 -1; 2 1]  RevolutionCrossSectionUnits=m  RevolutionExtent=Full  RevolutionAngle=180  RevolutionAngleUnits=deg
  To bottom black strip : sm_lib/Frames and Transforms/Rigid Transform  Commented=on  TranslationMethod=Cartesian  TranslationStandardOffset=0  TranslationLengthUnit=m  TranslationStandardAxis=+Z  TranslationCartesianOffset=[-xland/2, 0, 0]  TranslationROffset=0  TranslationROffsetUnits=m  TranslationZOffset=0  TranslationZOffsetUnits=m  TranslationThetaOffset=0  TranslationThetaOffsetUnits=deg  RotationMethod=None  RotationAngleUnits=deg  RotationStandardAxis=+Z  RotationAngle=0.0  RotationArbitraryAxis=[0 0 1]  FollAlignAxisA=+X  BaseAlignAxisA=+Y  FollAlignAxisB=+Y  BaseAlignAxisB=+Z  RotationSequenceAxes=FollowerAxes  RotationSequence=XYX  RotationSequenceAngles=[0 0 0]  RotationSequenceAnglesUnits=deg  RotationMatrix=[1 0 0; 0 1 0; 0 0 1]
  To left black strip : sm_lib/Frames and Transforms/Rigid Transform  Commented=on  TranslationMethod=Cartesian  TranslationStandardOffset=0  TranslationLengthUnit=m  TranslationStandardAxis=+Z  TranslationCartesianOffset=[0, yland/2, 0]  TranslationROffset=0  TranslationROffsetUnits=m  TranslationZOffset=0  TranslationZOffsetUnits=m  TranslationThetaOffset=0  TranslationThetaOffsetUnits=deg  RotationMethod=None  RotationAngleUnits=deg  RotationStandardAxis=+Z  RotationAngle=0.0  RotationArbitraryAxis=[0 0 1]  FollAlignAxisA=+X  BaseAlignAxisA=+Y  FollAlignAxisB=+Y  BaseAlignAxisB=+Z  RotationSequenceAxes=FollowerAxes  RotationSequence=XYX  RotationSequenceAngles=[0 0 0]  RotationSequenceAnglesUnits=deg  RotationMatrix=[1 0 0; 0 1 0; 0 0 1]
  To right black strip : sm_lib/Frames and Transforms/Rigid Transform  Commented=on  TranslationMethod=Cartesian  TranslationStandardOffset=0  TranslationLengthUnit=m  TranslationStandardAxis=+Z  TranslationCartesianOffset=[0, -yland/2, 0]  TranslationROffset=0  TranslationROffsetUnits=m  TranslationZOffset=0  TranslationZOffsetUnits=m  TranslationThetaOffset=0  TranslationThetaOffsetUnits=deg  RotationMethod=None  RotationAngleUnits=deg  RotationStandardAxis=+Z  RotationAngle=0.0  RotationArbitraryAxis=[0 0 1]  FollAlignAxisA=+X  BaseAlignAxisA=+Y  FollAlignAxisB=+Y  BaseAlignAxisB=+Z  RotationSequenceAxes=FollowerAxes  RotationSequence=XYX  RotationSequenceAngles=[0 0 0]  RotationSequenceAnglesUnits=deg  RotationMatrix=[1 0 0; 0 1 0; 0 0 1]
  To top black strip : sm_lib/Frames and Transforms/Rigid Transform  Commented=on  TranslationMethod=Cartesian  TranslationStandardOffset=0  TranslationLengthUnit=m  TranslationStandardAxis=+Z  TranslationCartesianOffset=[xland/10, 0, -0.1]  TranslationROffset=0  TranslationROffsetUnits=m  TranslationZOffset=0  TranslationZOffsetUnits=m  TranslationThetaOffset=0  TranslationThetaOffsetUnits=deg  RotationMethod=None  RotationAngleUnits=deg  RotationStandardAxis=+Z  RotationAngle=0.0  RotationArbitraryAxis=[0 0 1]  FollAlignAxisA=+X  BaseAlignAxisA=+Y  FollAlignAxisB=+Y  BaseAlignAxisB=+Z  RotationSequenceAxes=FollowerAxes  RotationSequence=XYX  RotationSequenceAngles=[0 0 0]  RotationSequenceAnglesUnits=deg  RotationMatrix=[1 0 0; 0 1 0; 0 0 1]
  Top black strip : sm_lib/Body Elements/Solid  Commented=on  InertiaType=CalculateFromGeometry  Mass=1  MassUnits=kg  CenterOfMass=[0 0 0]  CenterOfMassUnits=m  MomentsOfInertia=[1 1 1]  MomentsOfInertiaUnits=kg*m^2  ProductsOfInertia=[1 1 1]  ProductsOfInertiaUnits=kg*m^2  DensityBased=on  Density=1000  DensityUnits=kg/m^3  DoExposeReferenceFrame=on  SerializedFrames=<Frames/>  GraphicType=FromGeometry  MarkerShape=Sphere  MarkerSize=10  GraphicVisPropType=SimpleVisualProperties  GraphicDiffuseColor=[0.0 0.0 0.0]  GraphicSpecularColor=[0.5 0.5 0.5 1.0]  GraphicAmbientColor=[0.15 0.15 0.15 1.0]  GraphicEmissiveColor=[0.0 0.0 0.0 1.0]  GraphicShininess=75  GraphicOpacity=1.0  GeometryShape=Brick  RectangleSize=[1 1]  RectangleSizeUnits=m  BrickDimensions=[tblackstrip, yland, 0.1]  BrickDimensionUnits=m  CylinderRadius=1  CylinderRadiusUnits=m  CylinderLength=1  CylinderLengthUnits=m  SphereRadius=1  SphereRadiusUnits=m  EllipsoidRadii=[1 1 1]  EllipsoidRadiiUnits=m  ExtrusionCrossSection=[1 1; -1 1; -1 -1; 1 -1]  ExtrusionCrossSectionUnits=m  ExtrusionLength=1  ExtrusionLengthUnits=m  PolygonNumSides=3  PolygonOuterRadius=1  PolygonOuterRadiusUnits=m  ExtGeomFileType=STEP  ExtGeomFileUnits=m  RevolutionCrossSection=[1 1; 1 -1; 2 -1; 2 1]  RevolutionCrossSectionUnits=m  RevolutionExtent=Full  RevolutionAngle=180  RevolutionAngleUnits=deg
  Conn1 : PMIOPort  Port=1  Side=Left
  connections:
  Runway/RConn1 -- Rigid Transform/LConn1 -- To left black strip/LConn1 -- To right black strip/LConn1 -- To bottom black strip/LConn1 -- Conn1/RConn1
  Lane marker 1/RConn1 -- Rigid Transform1/LConn1 -- Rigid Transform/RConn1
  Lane marker 2/RConn1 -- Rigid Transform2/LConn1 -- Rigid Transform1/RConn1
  Lane marker 3/RConn1 -- Rigid Transform3/LConn1 -- Rigid Transform2/RConn1
  Lane marker 4/RConn1 -- Rigid Transform4/LConn1 -- Rigid Transform3/RConn1
  Rigid Transform7/LConn1 -- Top black strip/RConn1 -- To top black strip/RConn1
  Grass right of runway/RConn1 -- Rigid Transform6/RConn1
  Grass left of runway/RConn1 -- Rigid Transform5/RConn1
  Grass in front of runway/RConn1 -- Rigid Transform7/RConn1
  Grass behind runway/RConn1 -- Rigid Transform8/RConn1
  To top black strip/LConn1 -- Lane marker 5/RConn1 -- Rigid Transform4/RConn1
  Rigid Transform8/LConn1 -- Bottom black strip/RConn1 -- To bottom black strip/RConn1
  Rigid Transform6/LConn1 -- Right black strip/RConn1 -- To right black strip/RConn1
  Rigid Transform5/LConn1 -- Left black strip/RConn1 -- To left black strip/RConn1

== system AircraftSimulation_RealTime1a/Aircraft Simulation/Dynamics Simscape/Wind Disturbance/Wind Disturbance  ==
  Trigger : TriggerPort  VariantControl=Variant
  dV_Disturbance : Constant  Value="[dV_x;  dV_y;  dV_z]"
  Out1 : Outport  InitialOutput=[0; 0; 0]
  wires:
  dV_Disturbance/1 -> Out1/1

== system AircraftSimulation_RealTime1a/Aircraft Simulation/Flight Command/Command disturbance/Cmd Disturbance  ==
  Trigger : TriggerPort  VariantControl=Variant
  dV_Disturbance : Constant  Value="[dT;  de; da;  dr]"
  Out1 : Outport  InitialOutput=[0; 0; 0; 0]
  wires:
  dV_Disturbance/1 -> Out1/1

== system AircraftSimulation_RealTime1a/Aircraft Simulation/Dynamics Simscape/Derived States/Cannot Divide By Zero/Else Action Subsystem ==
  In1 : Inport
  Action Port : ActionPort  ActionType=else
  Out1 : Outport
  wires:
  In1/1 -> Out1/1

== system AircraftSimulation_RealTime1a/Aircraft Simulation/Dynamics Simscape/Derived States/Cannot Divide By Zero/If Action Subsystem  ==
  Action Port : ActionPort  ActionType=then
  Constant : Constant
  Out1 : Outport
  wires:
  Constant/1 -> Out1/1

== system AircraftSimulation_RealTime1a/Aircraft Simulation/Dynamics Simscape/Derived States/Cannot Divide By Zero1/Else Action Subsystem ==
  In1 : Inport
  Action Port : ActionPort  ActionType=else
  Out1 : Outport
  wires:
  In1/1 -> Out1/1

== system AircraftSimulation_RealTime1a/Aircraft Simulation/Dynamics Simscape/Derived States/Cannot Divide By Zero1/If Action Subsystem  ==
  Action Port : ActionPort  ActionType=then
  Constant : Constant
  Out1 : Outport
  wires:
  Constant/1 -> Out1/1

== matlab function AircraftSimulation_RealTime1a/Aircraft Simulation/Flight Command/Coordinated Turn ==
  data: T output; de output; da output; dr output; V input; TurnRate input; TurnAngle input; RoC input; TurnStates output; Constants input; AeroCoeffs input; LatControlMatrix input; LatKinematicMatrix input
function [T, de, da, dr, TurnStates] = fcn(V, TurnRate, TurnAngle, RoC, Constants, AeroCoeffs, LatControlMatrix, LatKinematicMatrix)
%#codegen

% LatControlMatrix = [CYB, CYda, CYdr; ClB, Clda, Cldr; CnB, Cnda, Cndr];
% LatKinematicMatrix = [CYp, CYr; Clp, Clr; Cnp, Cnr];

W = Constants(1);
rho = Constants(2);
AR = Constants(3);
S = Constants(4);
e = Constants(5);

CLo = AeroCoeffs(1,1);
CLa = AeroCoeffs(1,2);
CLde = AeroCoeffs(1,3);
CLq = AeroCoeffs(1,4);
Cmo = AeroCoeffs(2,1);
Cma = AeroCoeffs(2,2);
Cmde = AeroCoeffs(2,3);
Cmq = AeroCoeffs(2,4);
cdo = AeroCoeffs(3,1);

g = 9.81;
CLmax = Constants(6);
b = Constants(7);

% Turn analysis
TurnRate = TurnRate*pi/180;
ThetaTurn = RoC; % Climb angle during turn 

PhiTurn = atan(TurnRate*V/g);

TurnAngle = TurnAngle*pi/180; %rad
TimeTurn = TurnAngle/TurnRate; %s
n = 1/cos(PhiTurn); % load factor
Rturn=(2*W/(rho*g*S*CLmax))*(n/sqrt(n^2-1));

TurnControls = LatControlMatrix\LatKinematicMatrix*[sin(ThetaTurn); cos(ThetaTurn)*cos(PhiTurn)].*TurnRate*b./(2*V);

Beta = TurnControls(1)*180/pi;
da = TurnControls(2)*180/pi;
dr = TurnControls(3)*180/pi;

% Longitudinal stability analysis

Cw = W/(.5*rho*V^2*S);

Amat = [CLa CLde CLq; Cma Cmde Cmq];
Bmat = [n*Cw - CLo; -Cmo];
Trimmat = Amat\Bmat;

alphatrim = Trimmat(1);
etrim = Trimmat(2);
de = etrim;

CL = CLo + CLa*alphatrim + CLde*etrim;
CD = cdo + CL^2/(pi*e*AR);

T = 0.5*rho*V^2*S*CD;

TurnStates = [alphatrim*180/pi, Rturn, TimeTurn, n, Beta];

== matlab function AircraftSimulation_RealTime1a/Aircraft Simulation/Flight Command/MATLAB Function ==
  data: SteadyCmd input; Cmd output; TurnCmd input; ClimbCmd input; Steady input; Turn input; Climb input
function Cmd = fcn(SteadyCmd, TurnCmd, ClimbCmd, Steady, Turn, Climb)

if Turn == 1 && Climb == 1
    Cmd = TurnCmd;
    
elseif Steady == 1
    Cmd = SteadyCmd;
    
elseif Climb == 1
    Cmd = ClimbCmd;
    
elseif Turn == 1
    Cmd = TurnCmd;
    
else
    Cmd = SteadyCmd;
end

== matlab function AircraftSimulation_RealTime1a/Aircraft Simulation/Flight Command/Steady Level Flight  ==
  data: V input; InitialState output; Elevation input; Tcruise output; de output; da output; dr output; Constants input; AeroCoeffs input
function [InitialState, Tcruise, de, da, dr] = fcn(V, Elevation, Constants, AeroCoeffs)
%#codegen
W = Constants(1);
rho = Constants(2);
AR = Constants(3);
S = Constants(4);
e = Constants(5);

CLo = AeroCoeffs(1,1);
CLa = AeroCoeffs(1,2);
CLde = AeroCoeffs(1,3);
Cmo = AeroCoeffs(2,1);
Cma = AeroCoeffs(2,2);
Cmde = AeroCoeffs(2,3);
cdo = AeroCoeffs(3,1);

Cw = W/(.5*rho*V^2*S);

Amat = [CLa CLde;Cma Cmde];
Bmat = [Cw - CLo;-Cmo];
Trimmat = Amat\Bmat;

alphatrim = Trimmat(1);
etrim = Trimmat(2);
de = etrim;
da = 0;
dr = 0;

CL = CLo + CLa*alphatrim + CLde*etrim;
Cm = Cmo + Cma*alphatrim + Cmde*etrim;
CD = cdo + CL^2/(pi*e*AR);

Tcruise = 0.5*rho*V^2*S*CD;

u = V*cos(alphatrim);
w = V*sin(alphatrim);
v = 0;

vi = [u, v, w];

g = 9.81;
mu_e = 3.986004418*10^14;
r = sqrt(mu_e/g);
zi = r - Elevation; % Sea level altitude from center of Earth

xi = [0, 0, -zi];

% angi = [0 alphatrim 0];
angi = [0 0 0];
omgi = [0 0 0];

InitialState = zeros(4,3);
InitialState(1,:) = xi;
InitialState(2,:) = vi;
InitialState(3,:) = angi;
InitialState(4,:) = omgi;

== matlab function AircraftSimulation_RealTime1a/Aircraft Simulation/Dynamics Simscape/Quaternion to Euler ==
  data: q input; angles output; out output
function [angles, out] = fcn(q)

q0 = q(1);
q1 = q(2);
q2 = q(3);
q3 = q(4);

phi   = atan2(2*(q0*q1+q2*q3),1-2*(q1^2+q2^2));
if q2 > q0
    theta = pi - asin(2*(q0*q2-q3*q1));
    out = 1;
else
theta = asin(2*(q0*q2-q3*q1));
out = 0;
end
psi   = atan2(2*(q0*q3+q1*q2),1-2*(q2^2+q3^2));

angles = [phi, theta, psi];
